simulink model "junction_loop_2018a"  (R2018a)
settings: Solver=FixedStepDiscrete  StartTime=0.0  StopTime=0.1  FixedStep=0.1  RelTol=1e-3  EnableMultiTasking=on
settings Model: Creator=BEAR  LastModifiedBy=bzhan
settings SolverCC: AutoInsertRateTranBlk=on
settings DataIOCC: LimitDataPoints=on
settings OptimizationCC: LifeSpan=inf
settings DebuggingCC: AllowSymbolicDim=off  SFUnexpectedBacktrackingDiag=warning  SFNoUnconditionalDefaultTransitionDiag=warning  SFExecutionAtInitializationDiag=none
settings CodeAppCC: StateflowObjectComments=on
settings GRTTargetCC: TargetLangStandard=C89/C90 (ANSI)
settings ConfigComp: CovMetricSettings=dw  CovHtmlReporting=on  CovSaveCumulativeToWorkspaceVar=on  CovSaveSingleToWorkspaceVar=on  CovShowResultsExplorer=off  CovExternalEMLEnable=off  CovSFcnEnable=off

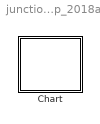
== system junction_loop_2018a ==
  Chart : Stateflow chart  TreatAsAtomicUnit=on

== stateflow chart junction_loop_2018a/Chart ==
  state A
  state B
  (junction 5) -> A [order 1] : [x==1]{f("t4")}
  (default) -> A : {x=5}
  (junction 4) -> (junction 5) : {x=x-1;f("t1")}
  A -> (junction 4)
  (junction 5) -> B [order 3] : {f("t3")}
  (junction 5) -> (junction 4) [order 2] : [x>0]{f("t2")}
  data: s function_input; x local
  function f(s):
    | function f(s)
    |   fprintf(s+"\n");
